simulink model "M1_P3_B_2"  (R2023a)
settings: Solver=VariableStepAuto  StartTime=0.0  StopTime=2.5  RelTol=1e-3
undefined symbols (not defined in the file): f_eff, J_eff, Kb, Ktn, L, P, R
settings Model: Creator=azzam  LastModifiedBy=azzam

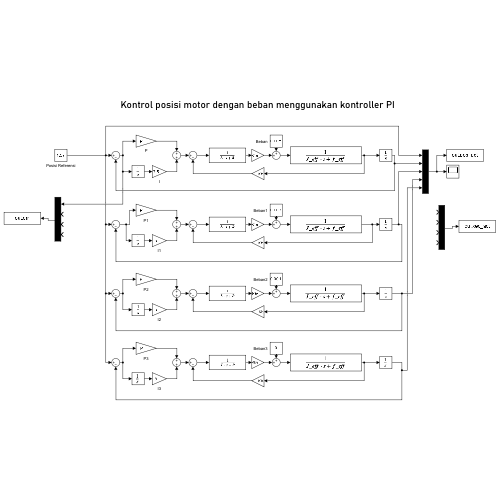
[thumbnail: Simulink's stored preview of the top-level diagram]
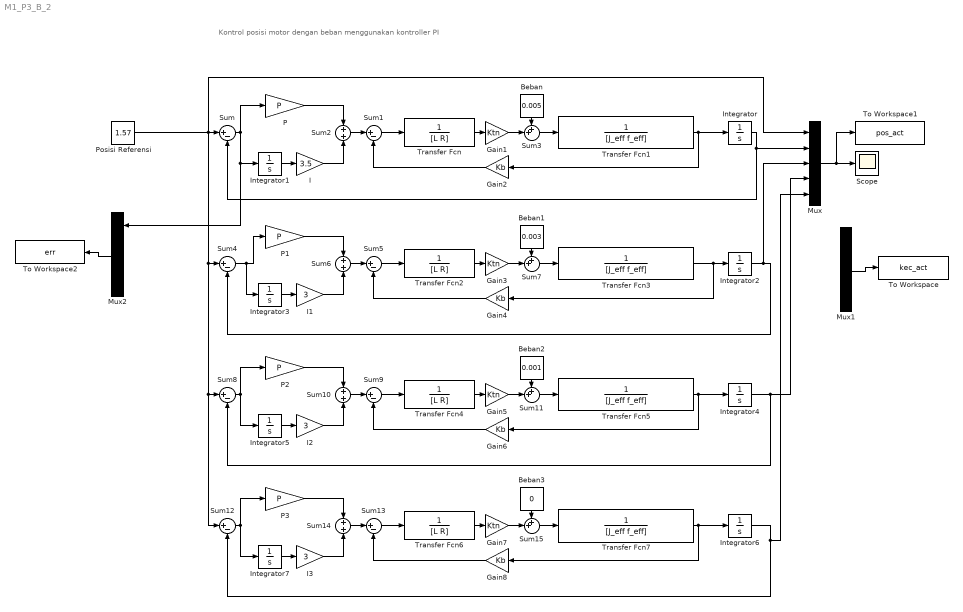
== system M1_P3_B_2 ==
  note: Kontrol posisi motor dengan beban menggunakan kontroller PI
  Beban : Constant  Value=0.005
  Beban1 : Constant  Value=0.003
  Beban2 : Constant  Value=0.001
  Beban3 : Constant  Value=0
  Gain{1,3,5,7} (4 alike) : Gain  Gain=Ktn
  Gain{2,4,6,8} (4 alike) : Gain  Gain=Kb
  I : Gain  Gain=3.5
  I1 : Gain  Gain=3
  I2 : Gain  Gain=3
  I3 : Gain  Gain=3
  Integrator{,1..7} (8 alike) : Integrator
  Mux : Mux  Inputs=5
  Mux1 : Mux
  Mux2 : Mux
  P{,1..3} (4 alike) : Gain  Gain=P
  Posisi Referensi : Constant  Value=1.57
  Scope : Scope
  Sum{,1,4..5,8..9,12..13} (8 alike) : Sum  Inputs=|+-
  Sum{2,6,10,14} (4 alike) : Sum
  Sum{3,7,11,15} (4 alike) : Sum  Inputs=++|
  To Workspace : ToWorkspace  VariableName=kec_act  SaveFormat=Timeseries  SampleTime=-1
  To Workspace1 : ToWorkspace  VariableName=pos_act  SaveFormat=Timeseries  SampleTime=-1
  To Workspace2 : ToWorkspace  VariableName=err  SaveFormat=Timeseries  SampleTime=-1
  Transfer Fcn{,2,4,6} (4 alike) : TransferFcn  Denominator=[L R]
  Transfer Fcn{1,3,5,7} (4 alike) : TransferFcn  Denominator=[J_eff f_eff]
  wires:
  Mux1/1 -> To Workspace/1
  Integrator/1 -> Sum/2, Mux/2
  Transfer Fcn1/1 -> Gain2/1, Integrator/1
  Transfer Fcn/1 -> Gain1/1
  Sum/1 -> Integrator1/1, Mux2/1, P/1
  Gain2/1 -> Sum1/2
  Sum1/1 -> Transfer Fcn/1
  Mux/1 -> To Workspace1/1, Scope/1
  Mux2/1 -> To Workspace2/1
  Sum2/1 -> Sum1/1
  P/1 -> Sum2/1
  I/1 -> Sum2/2
  Integrator1/1 -> I/1
  Gain1/1 -> Sum3/2
  Sum3/1 -> Transfer Fcn1/1
  Beban/1 -> Sum3/1
  Sum5/1 -> Transfer Fcn2/1
  Integrator2/1 -> Mux/3, Sum4/2
  Sum4/1 -> Integrator3/1, P1/1
  P1/1 -> Sum6/1
  Transfer Fcn2/1 -> Gain3/1
  Sum6/1 -> Sum5/1
  Integrator3/1 -> I1/1
  Gain4/1 -> Sum5/2
  I1/1 -> Sum6/2
  Transfer Fcn3/1 -> Gain4/1, Integrator2/1
  Sum7/1 -> Transfer Fcn3/1
  Gain3/1 -> Sum7/2
  Beban1/1 -> Sum7/1
  Integrator4/1 -> Mux/4, Sum8/2
  Beban2/1 -> Sum11/1
  Gain5/1 -> Sum11/2
  Integrator5/1 -> I2/1
  Transfer Fcn5/1 -> Gain6/1, Integrator4/1
  Gain6/1 -> Sum9/2
  I2/1 -> Sum10/2
  Sum11/1 -> Transfer Fcn5/1
  Sum10/1 -> Sum9/1
  Transfer Fcn4/1 -> Gain5/1
  Sum8/1 -> Integrator5/1, P2/1
  P2/1 -> Sum10/1
  Sum9/1 -> Transfer Fcn4/1
  Integrator6/1 -> Mux/5, Sum12/2
  Beban3/1 -> Sum15/1
  Gain7/1 -> Sum15/2
  Integrator7/1 -> I3/1
  Transfer Fcn7/1 -> Gain8/1, Integrator6/1
  Gain8/1 -> Sum13/2
  I3/1 -> Sum14/2
  Sum15/1 -> Transfer Fcn7/1
  Sum14/1 -> Sum13/1
  Transfer Fcn6/1 -> Gain7/1
  Sum12/1 -> Integrator7/1, P3/1
  P3/1 -> Sum14/1
  Sum13/1 -> Transfer Fcn6/1
  Posisi Referensi/1 -> Sum4/1, Sum8/1, Sum12/1, Mux/1, Sum/1
